simulink model "WT_modelv2"  (R2015a)
settings: Solver=ode3  StartTime=0.0  StopTime=3  FixedStep=Ts  RelTol=1e-3
values from neighbouring files (symbols this model uses):
  Ka = fluxeff    (= 0.15)    [VOC_param.m]    (also in VOC_param_paper.m; power_control_param.m)
  Ls = 2.7e-3    (= 0.0027)    [power_control_param.m]
  p = 4    [VOC_param.m]    (also in VOC_param_paper.m; power_control_param.m)
  rpm2radps = pi/30    (= 0.10471975512)    [VOC_param.m]    (also in VOC_param_paper.m; power_control_param.m)
  Rs = 1.137    [power_control_param.m]
settings Model: Creator=rblan  LastModifiedBy=rblan

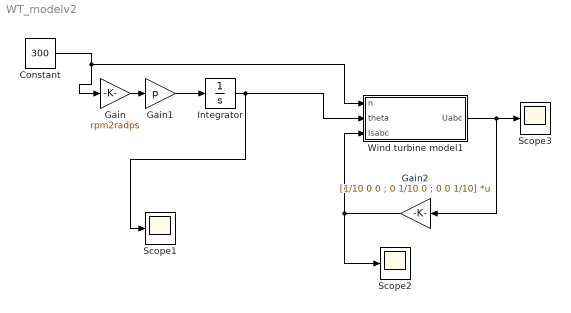
== system WT_modelv2 ==
  Constant : Constant  Value=300
  Gain : Gain  Gain=rpm2radps
  Gain1 : Gain  Gain=p
  Gain2 : Gain  Gain=[1/10 0 0 ; 0 1/10 0 ; 0 0 1/10]  Multiplication=Matrix(K*u)
  Integrator : Integrator
  Scope1 : Scope
      settings: YMin=-400  YMax=400  SaveName=ScopeData3
  Scope2 : Scope
      settings: YMin=-1.75  YMax=1.75  SaveName=ScopeData5
  Scope3 : Scope
      settings: YMin=-17.5  YMax=17.5
  Wind turbine model1 : Subsystem
  wires:
  Wind turbine model1/1(Uabc) -> Gain2/1, Scope3/1
  Constant/1 -> Wind turbine model1/1(n), Gain/1
  Gain/1 -> Gain1/1
  Integrator/1 -> Scope1/1, Wind turbine model1/2(theta)
  Gain1/1 -> Integrator/1
  Gain2/1 -> Wind turbine model1/3(Isabc), Scope2/1

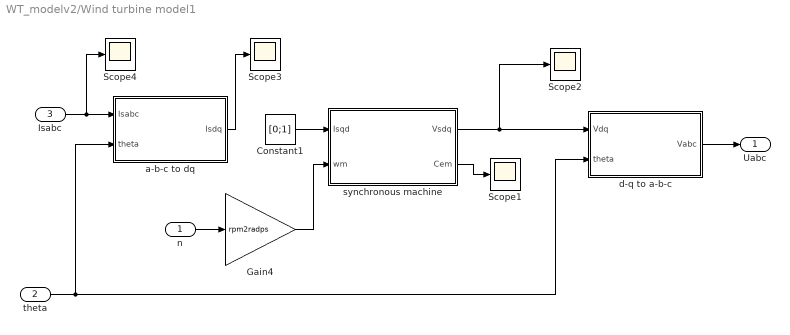
== system WT_modelv2/Wind turbine model1 ==
  n : Inport
  theta : Inport  Port=2
  Isabc : Inport  Port=3
  Constant1 : Constant  Value=[0;1]
  Gain4 : Gain  Gain=rpm2radps
  Scope{1..4} (4 alike) : Scope
      Scope2 settings: YMin=-1  YMax=20  SaveName=ScopeData4
      Scope3 settings: YMin=-0.1  YMax=2.2  SaveName=ScopeData2
      Scope4 settings: YMin=-0.7  YMax=1.3  SaveName=ScopeData6
  a-b-c to dq : Subsystem
  d-q to a-b-c : Subsystem
  synchronous machine : Subsystem
  Uabc : Outport
  wires:
  synchronous machine/2(Cem) -> Scope1/1
  synchronous machine/1(Vsdq) -> Scope2/1, d-q to a-b-c/1(Vdq)
  d-q to a-b-c/1(Vabc) -> Uabc/1
  theta/1 -> d-q to a-b-c/2(theta), a-b-c to dq/2(theta)
  a-b-c to dq/1(Isdq) -> Scope3/1
  Isabc/1 -> Scope4/1, a-b-c to dq/1(Isabc)
  Gain4/1 -> synchronous machine/2(wm)
  n/1 -> Gain4/1
  Constant1/1 -> synchronous machine/1(Isqd)

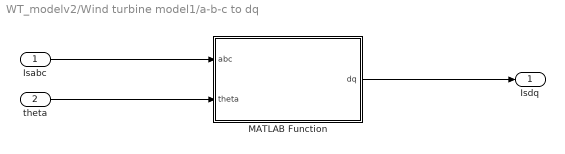
== system WT_modelv2/Wind turbine model1/a-b-c to dq ==
  Isabc : Inport
  theta : Inport  Port=2
  MATLAB Function : MATLAB Function  TreatAsAtomicUnit=on
  Isdq : Outport
  wires:
  Isabc/1 -> MATLAB Function/1(abc)
  theta/1 -> MATLAB Function/2(theta)
  MATLAB Function/1(dq) -> Isdq/1

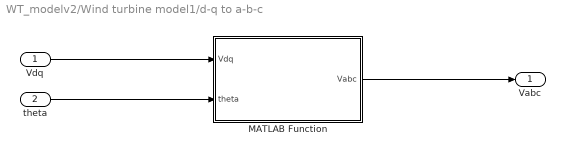
== system WT_modelv2/Wind turbine model1/d-q to a-b-c ==
  Vdq : Inport
  theta : Inport  Port=2
  MATLAB Function : MATLAB Function  TreatAsAtomicUnit=on
  Vabc : Outport
  wires:
  Vdq/1 -> MATLAB Function/1(Vdq)
  theta/1 -> MATLAB Function/2(theta)
  MATLAB Function/1(Vabc) -> Vabc/1

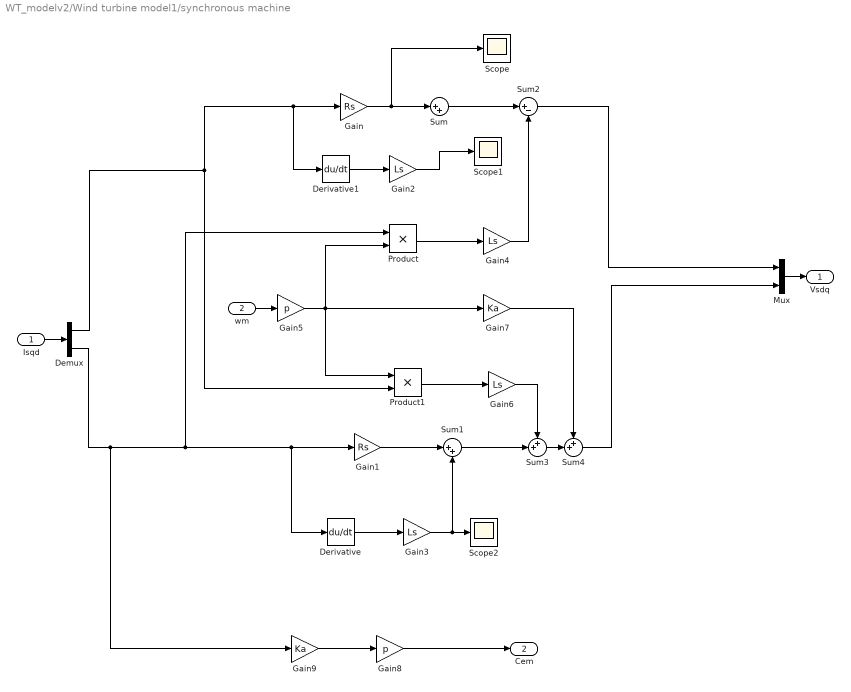
== system WT_modelv2/Wind turbine model1/synchronous machine ==
  Isqd : Inport
  wm : Inport  Port=2
  Demux : Demux  Outputs=2
  Derivative : Derivative
  Derivative1 : Derivative
  Gain : Gain  Gain=Rs
  Gain1 : Gain  Gain=Rs
  Gain{2..4,6} (4 alike) : Gain  Gain=Ls
  Gain5 : Gain  Gain=p
  Gain7 : Gain  Gain=Ka
  Gain8 : Gain  Gain=p
  Gain9 : Gain  Gain=Ka
  Mux : Mux  Inputs=2
  Product : Product
  Product1 : Product
  Scope : Scope
      settings: SaveName=ScopeData7
  Scope1 : Scope
      settings: SaveName=ScopeData8
  Scope2 : Scope
      settings: SaveName=ScopeData9
  Sum : Sum  Inputs=|++
  Sum1 : Sum  Inputs=|++
  Sum2 : Sum  Inputs=|+-
  Sum3 : Sum  Inputs=++|
  Sum4 : Sum  Inputs=++|
  Vsdq : Outport
  Cem : Outport  Port=2
  wires:
  Demux/1 -> Product1/2, Derivative1/1, Gain/1
  Demux/2 -> Derivative/1, Gain1/1, Product/1, Gain9/1
  Gain/1 -> Scope/1, Sum/1
  Derivative1/1 -> Gain2/1
  Gain2/1 -> Scope1/1
  Derivative/1 -> Gain3/1
  wm/1 -> Gain5/1
  Product/1 -> Gain4/1
  Gain4/1 -> Sum2/2
  Gain6/1 -> Sum3/1
  Product1/1 -> Gain6/1
  Gain5/1 -> Product1/1, Gain7/1, Product/2
  Sum3/1 -> Sum4/2
  Gain7/1 -> Sum4/1
  Sum2/1 -> Mux/1
  Sum4/1 -> Mux/2
  Gain8/1 -> Cem/1
  Gain9/1 -> Gain8/1
  Mux/1 -> Vsdq/1
  Isqd/1 -> Demux/1
  Gain1/1 -> Sum1/1
  Sum/1 -> Sum2/1
  Sum1/1 -> Sum3/2
  Gain3/1 -> Sum1/2, Scope2/1

== matlab function WT_modelv2/Wind turbine model1/a-b-c to dq/MATLAB Function ==
  data: abc input; dq output; theta input
function dq = abc2dq(abc,theta)
% transformation from d-q to a-b-c
% based on "COMMANDE VECTORIELLE DES MACHINES ASYNCHRONES & SYNCHRONES" 
% 5ème Année GE Option ISIP INSA LYON
% http://docinsa.insa-lyon.fr/polycop/download.php?id=160503&id2=0 



dq=zeros(2,1) ; 
a= abc(1) ; 
b= abc(2) ; 
c=abc(3) ; 

d = cos(theta)*a + cos(theta-2*pi/3)*b + cos(theta+2*pi/3)*c ; 
q = -sin(theta)*a -sin(theta-2*pi/3)*b - sin(theta+2*pi/3)*c ; 

dq(1)=d ; 
dq(2)=q ; 


dq = sqrt(2/3) * dq ;

== matlab function WT_modelv2/Wind turbine model1/d-q to a-b-c/MATLAB Function ==
  data: Vdq input; Vabc output; theta input
function Vabc = fcn(Vdq,theta)
% transformation from d-q to a-b-c
% based on "COMMANDE VECTORIELLE DES MACHINES ASYNCHRONES & SYNCHRONES" 
% 5ème Année GE Option ISIP INSA LYON
% http://docinsa.insa-lyon.fr/polycop/download.php?id=160503&id2=0 



Vabc=zeros(3,1) ; 

Va = cos (theta)*Vdq(1) -sin(theta)*Vdq(2) ; 
Vb = cos(theta-2*pi/3)*Vdq(1) - sin(theta -2*pi/3)*Vdq(2) ; 
Vc = cos(theta+2*pi/3)*Vdq(1) - sin(theta+2*pi/3)*Vdq(2) ; 

Vabc(1)=Va ; 
Vabc(2)=Vb ; 
Vabc(3)=Vc ; 

Vabc = sqrt(2/3) * Vabc ;
